simulink model "Block"  (R2017a)
settings: Solver=VariableStepAuto  StartTime=0.0  StopTime=Tsim  FixedStep=0.0001  RelTol=1e-3
values from neighbouring files (symbols this model uses):
  b = 0.1    [Model_old.m]
  g = 40    [Model_old.m]    (also in ModeloBase_OLD.m)
  J = 0.01    [Model_old.m]
  Kd = 0    [Model_old.m]
  Ke = 0.08    [Model_old.m]
  Ki = 10.0    (= 10)    [Model_old.m]
  Kp = 5.0    (= 5)    [Model_old.m]
  ksi = 0.6    [Model_old.m]    (also in ModeloBase_OLD.m = 0.3)
  L = 0.5    [Model_old.m]
  R = 1    [Model_old.m]
  Ts = 0.1    [Model_old.m]    (also in ModeloBase_OLD.m; PIController.m)
undefined symbols (not defined in the file or in its folder): DiscIntNeverNeededParam, F_M
libraries: simulink x16, simulink_extras x2
settings Model: Creator=davi2  LastModifiedBy=davi2

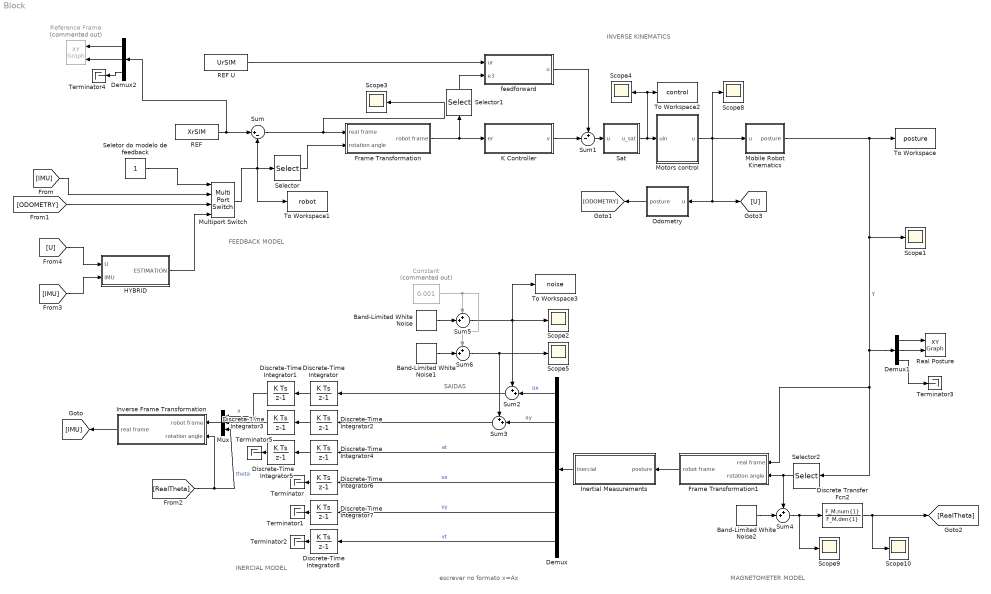
== system Block ==
  note: escrever no formato x=Ax
  note: SAIDAS
  note: INVERSE KINEMATICS
  note: MAGNETOMETER MODEL
  note: INERCIAL MODEL
  note: FEEDBACK MODEL
  Band-Limited White Noise : simulink/Sources/Band-Limited White Noise  Cov=0.000008  Ts=1/200  seed=[23341]
  Band-Limited White Noise1 : simulink/Sources/Band-Limited White Noise  Cov=0.000008  Ts=1/200  seed=[23341]
  Band-Limited White Noise2 : simulink/Sources/Band-Limited White Noise  Cov=0.00001  Ts=1/200  seed=[23341]
  Constant : Constant  Commented=on  Value=0.001
  Demux : Demux  Outputs=6
  Demux1 : Demux  Outputs=3
  Demux2 : Demux  Outputs=3
  Discrete Transfer Fcn2 : DiscreteTransferFcn  Numerator=F_M.num{1}  Denominator=F_M.den{1}
  Discrete-Time Integrator{,1..8} (9 alike) : DiscreteIntegrator  InitialConditionSetting=State (most efficient)  SampleTime=Ts  ICPrevOutput=DiscIntNeverNeededParam  ICPrevScaledInput=DiscIntNeverNeededParam
  Frame Transformation : Subsystem
  Frame Transformation1 : Subsystem
  HYBRID : Subsystem
  Inertial Measurements : Subsystem
  Inverse Frame Transformation : Subsystem
  K Controller : Subsystem
  Mobile Robot Kinematics : Subsystem
  Motors control : Subsystem
  Multiport Switch : MultiPortSwitch
  Mux : Mux  Inputs=3
  Odometry : Subsystem
  REF : FromWorkspace  VariableName=XrSIM  SampleTime=Ts  OutputAfterFinalValue=Holding final value
  REF U : FromWorkspace  VariableName=UrSIM  SampleTime=Ts  OutputAfterFinalValue=Holding final value
  Real Posture : simulink/Sinks/XY Graph  xmin=0  xmax=3  ymin=-0.8  ymax=1.5  st=Ts
  Reference Frame : simulink/Sinks/XY Graph  Commented=on  xmin=0  xmax=2  ymin=0  ymax=1.5  st=Ts
  Sat : Subsystem
  Scope{1..5,8..10} (8 alike) : Scope
  Selector : Selector  InputPortWidth=3  IndexOptions=Index vector (dialog)  Indices=3  OutputSizes=1
  Selector1 : Selector  InputPortWidth=3  IndexOptions=Index vector (dialog)  Indices=3  OutputSizes=1
  Selector2 : Selector  InputPortWidth=3  IndexOptions=Index vector (dialog)  Indices=3  OutputSizes=1
  Seletor do modelo de feedback : Constant
  Sum : Sum  Inputs=|+-
  Sum1 : Sum  Inputs=+-|
  Sum{2..6} (5 alike) : Sum  Inputs=++|
  Terminator{,1..5} (6 alike) : Terminator
  To Workspace : ToWorkspace  VariableName=posture  SaveFormat=Timeseries  SampleTime=-1
  To Workspace1 : ToWorkspace  VariableName=robot  SaveFormat=Timeseries  SampleTime=-1
  To Workspace2 : ToWorkspace  VariableName=control  SaveFormat=Timeseries  SampleTime=-1
  To Workspace3 : ToWorkspace  VariableName=noise  SaveFormat=Timeseries  SampleTime=-1
  feedforward : Subsystem
  wires:
  Sum/1 -> Scope3/1, Frame Transformation/1(real frame)
  Selector/1 -> Frame Transformation/2(rotation angle)
  Frame Transformation/1(robot frame) -> K Controller/1(er), Selector1/1
  REF U/1 -> feedforward/1(ur)
  Selector1/1 -> feedforward/2(e3)
  feedforward/1(u) -> Sum1/1
  K Controller/1(v) -> Sum1/2
  Motors control/1(u) -> Mobile Robot Kinematics/1(u), Scope8/1, Odometry/1(u), [U]
  Selector2/1 -> Frame Transformation1/2(rotation angle), Sum4/1
  Inertial Measurements/1(inercial) -> Demux/1
  Discrete-Time Integrator/1 -> Discrete-Time Integrator1/1
  Frame Transformation1/1(robot frame) -> Inertial Measurements/1(posture)
  Discrete-Time Integrator2/1 -> Discrete-Time Integrator3/1
  Discrete-Time Integrator4/1 -> Discrete-Time Integrator5/1
  Demux/4 -> Discrete-Time Integrator6/1  "vx"
  Demux/5 -> Discrete-Time Integrator7/1  "vy"
  Demux/6 -> Discrete-Time Integrator8/1  "vt"
  Discrete-Time Integrator1/1 -> Mux/1  "x"
  Discrete-Time Integrator3/1 -> Mux/2  "y"
  Mux/1 -> Inverse Frame Transformation/1(robot frame)
  Demux/1 -> Sum2/2  "ax"
  Demux1/1 -> Real Posture/1
  Demux1/2 -> Real Posture/2
  REF/1 -> Demux2/1, Sum/1
  Inverse Frame Transformation/1(real frame) -> [IMU]
  [IMU] -> Multiport Switch/2
  [ODOMETRY] -> Multiport Switch/3
  Odometry/1(posture) -> [ODOMETRY]
  Mobile Robot Kinematics/1(posture) -> To Workspace/1, Scope1/1, Demux1/1, Frame Transformation1/1(real frame), Selector2/1  "Y"
  Demux/3 -> Discrete-Time Integrator4/1  "at"
  Demux/2 -> Sum3/2  "ay"
  [RealTheta] -> Mux/3, Inverse Frame Transformation/2(rotation angle)  "theta"
  Sum2/1 -> Discrete-Time Integrator/1
  Sum3/1 -> Discrete-Time Integrator2/1
  Band-Limited White Noise/1 -> Sum5/2
  Sum5/1 -> To Workspace3/1, Scope2/1, Sum2/1
  Band-Limited White Noise1/1 -> Sum6/2
  Sum6/1 -> Scope5/1, Sum3/1
  Sum1/1 -> Sat/1(u)
  Sat/1(u_sat) -> Scope4/1, To Workspace2/1, Motors control/1(uin)
  Constant/1 -> Sum5/1, Sum6/1
  Multiport Switch/1 -> Sum/2, Selector/1, To Workspace1/1
  Discrete-Time Integrator6/1 -> Terminator/1
  Discrete-Time Integrator7/1 -> Terminator1/1
  Discrete-Time Integrator8/1 -> Terminator2/1
  Demux1/3 -> Terminator3/1
  Seletor do modelo de feedback/1 -> Multiport Switch/1
  Discrete-Time Integrator5/1 -> Terminator5/1
  HYBRID/1(ESTIMATION) -> Multiport Switch/4
  [IMU] -> HYBRID/2(IMU)
  [U] -> HYBRID/1(U)
  Band-Limited White Noise2/1 -> Sum4/2
  Sum4/1 -> Discrete Transfer Fcn2/1, Scope9/1
  Discrete Transfer Fcn2/1 -> [RealTheta], Scope10/1
  Demux2/1 -> Reference Frame/1
  Demux2/2 -> Reference Frame/2
  Demux2/3 -> Terminator4/1

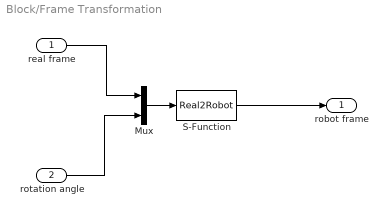
== system Block/Frame Transformation ==
  real frame : Inport
  rotation angle : Inport  Port=2
  Mux : Mux  Inputs=2
  S-Function : S-Function  FunctionName=Real2Robot  Parameters=Ts  SFunctionDeploymentMode=off  EnableBusSupport=off
  robot frame : Outport
  wires:
  real frame/1 -> Mux/1
  rotation angle/1 -> Mux/2
  Mux/1 -> S-Function/1
  S-Function/1 -> robot frame/1

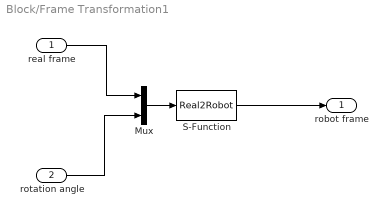
== system Block/Frame Transformation1 ==
  real frame : Inport
  rotation angle : Inport  Port=2
  Mux : Mux  Inputs=2
  S-Function : S-Function  FunctionName=Real2Robot  Parameters=Ts  SFunctionDeploymentMode=off  EnableBusSupport=off
  robot frame : Outport
  wires:
  real frame/1 -> Mux/1
  rotation angle/1 -> Mux/2
  Mux/1 -> S-Function/1
  S-Function/1 -> robot frame/1

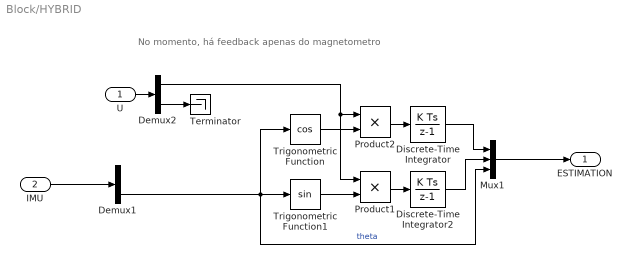
== system Block/HYBRID ==
  note: No momento, há feedback apenas do magnetometro
  U : Inport
  IMU : Inport  Port=2
  Demux1 : Demux  Outputs=3
  Demux2 : Demux  Outputs=2
  Discrete-Time Integrator : DiscreteIntegrator  InitialConditionSetting=State (most efficient)  SampleTime=Ts  ICPrevOutput=DiscIntNeverNeededParam  ICPrevScaledInput=DiscIntNeverNeededParam
  Discrete-Time Integrator2 : DiscreteIntegrator  InitialConditionSetting=State (most efficient)  SampleTime=Ts  ICPrevOutput=DiscIntNeverNeededParam  ICPrevScaledInput=DiscIntNeverNeededParam
  Mux1 : Mux  Inputs=3
  Product1 : Product
  Product2 : Product
  Terminator : Terminator
  Trigonometric Function : Trigonometry  Operator=cos
  Trigonometric Function1 : Trigonometry
  ESTIMATION : Outport
  wires:
  IMU/1 -> Demux1/1
  Trigonometric Function1/1 -> Product1/2
  Demux2/1 -> Product1/1, Product2/1
  Trigonometric Function/1 -> Product2/2
  Product2/1 -> Discrete-Time Integrator/1
  Discrete-Time Integrator/1 -> Mux1/1
  Discrete-Time Integrator2/1 -> Mux1/2
  Demux1/3 -> Mux1/3, Trigonometric Function/1, Trigonometric Function1/1  "theta"
  Product1/1 -> Discrete-Time Integrator2/1
  Mux1/1 -> ESTIMATION/1
  U/1 -> Demux2/1
  Demux2/2 -> Terminator/1

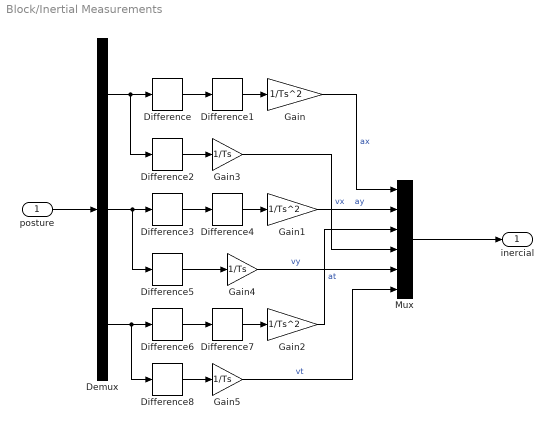
== system Block/Inertial Measurements ==
  posture : Inport
  Demux : Demux  Outputs=3
  Difference{,1..8} (9 alike) : simulink/Discrete/Difference  ICPrevInput=0.0  OutMin=[]  OutMax=[]  OutDataType=fixdt(1, 16)  OutScaling=2^-10  DoSatur=off
  Gain : Gain  Gain=1/Ts^2
  Gain1 : Gain  Gain=1/Ts^2
  Gain2 : Gain  Gain=1/Ts^2
  Gain3 : Gain  Gain=1/Ts
  Gain4 : Gain  Gain=1/Ts
  Gain5 : Gain  Gain=1/Ts
  Mux : Mux  Inputs=6
  inercial : Outport
  wires:
  posture/1 -> Demux/1
  Difference/1 -> Difference1/1
  Difference3/1 -> Difference4/1
  Difference6/1 -> Difference7/1
  Demux/3 -> Difference8/1, Difference6/1
  Demux/2 -> Difference5/1, Difference3/1
  Demux/1 -> Difference2/1, Difference/1
  Difference1/1 -> Gain/1
  Difference4/1 -> Gain1/1
  Difference7/1 -> Gain2/1
  Gain2/1 -> Mux/3  "at"
  Gain1/1 -> Mux/2  "ay"
  Gain/1 -> Mux/1  "ax"
  Difference2/1 -> Gain3/1
  Difference8/1 -> Gain5/1
  Difference5/1 -> Gain4/1
  Gain3/1 -> Mux/4  "vx"
  Gain4/1 -> Mux/5  "vy"
  Gain5/1 -> Mux/6  "vt"
  Mux/1 -> inercial/1

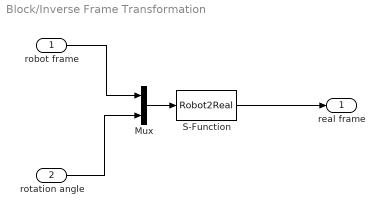
== system Block/Inverse Frame Transformation ==
  robot frame : Inport
  rotation angle : Inport  Port=2
  Mux : Mux  Inputs=2
  S-Function : S-Function  FunctionName=Robot2Real  Parameters=Ts  SFunctionDeploymentMode=off  EnableBusSupport=off
  real frame : Outport
  wires:
  robot frame/1 -> Mux/1
  rotation angle/1 -> Mux/2
  Mux/1 -> S-Function/1
  S-Function/1 -> real frame/1

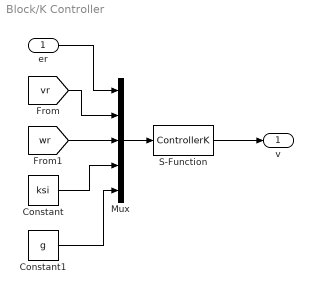
== system Block/K Controller ==
  er : Inport
  Constant : Constant  Value=ksi
  Constant1 : Constant  Value=g
  Mux : Mux  Inputs=5
  S-Function : S-Function  FunctionName=ControllerK  Parameters=Ts  SFunctionDeploymentMode=off  EnableBusSupport=off
  v : Outport
  wires:
  er/1 -> Mux/1
  [vr] -> Mux/2
  [wr] -> Mux/3
  Constant/1 -> Mux/4
  Constant1/1 -> Mux/5
  Mux/1 -> S-Function/1
  S-Function/1 -> v/1

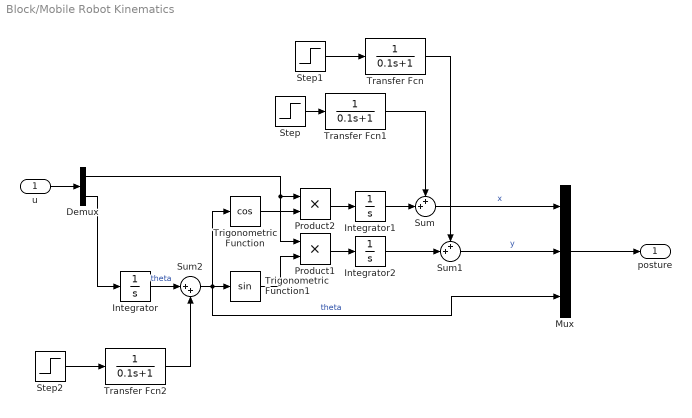
== system Block/Mobile Robot Kinematics ==
  u : Inport
  Demux : Demux  Outputs=2
  Integrator : Integrator
  Integrator1 : Integrator
  Integrator2 : Integrator
  Mux : Mux  Inputs=3
  Product1 : Product
  Product2 : Product
  Step : Step  Time=20  After=0.5  SampleTime=0
  Step1 : Step  Time=10  After=-0.5  SampleTime=0
  Step2 : Step  Time=5  After=0  SampleTime=0
  Sum : Sum  Inputs=++|
  Sum1 : Sum  Inputs=++|
  Sum2 : Sum  Inputs=|++
  Transfer Fcn : TransferFcn  Denominator=[0.1 1]
  Transfer Fcn1 : TransferFcn  Denominator=[0.1 1]
  Transfer Fcn2 : TransferFcn  Denominator=[0.1 1]
  Trigonometric Function : Trigonometry  Operator=cos
  Trigonometric Function1 : Trigonometry
  posture : Outport
  wires:
  u/1 -> Demux/1
  Demux/2 -> Integrator/1
  Trigonometric Function/1 -> Product2/2
  Demux/1 -> Product1/1, Product2/1
  Product2/1 -> Integrator1/1
  Trigonometric Function1/1 -> Product1/2
  Product1/1 -> Integrator2/1
  Mux/1 -> posture/1
  Transfer Fcn1/1 -> Sum/1
  Transfer Fcn/1 -> Sum1/1
  Step2/1 -> Transfer Fcn2/1
  Step1/1 -> Transfer Fcn/1
  Step/1 -> Transfer Fcn1/1
  Integrator1/1 -> Sum/2
  Integrator2/1 -> Sum1/2
  Sum/1 -> Mux/1  "x"
  Sum1/1 -> Mux/2  "y"
  Integrator/1 -> Sum2/1  "theta"
  Sum2/1 -> Trigonometric Function/1, Mux/3, Trigonometric Function1/1  "theta"
  Transfer Fcn2/1 -> Sum2/2

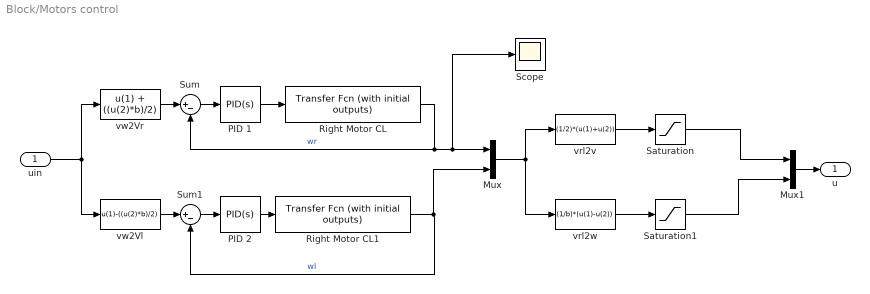
== system Block/Motors control ==
  uin : Inport
  Mux : Mux  Inputs=2
  Mux1 : Mux  Inputs=2
  PID 1 : simulink/Continuous/PID Controller  Controller=PID  TimeDomain=Continuous-time  SampleTime=-1  IntegratorMethod=Forward Euler  FilterMethod=Forward Euler  Form=Parallel  UseFilter=on  ControllerParametersSource=internal  P=Kp  I=Ki  D=Kd  N=100  InitialConditionSource=internal  InitialConditionForIntegrator=0  InitialConditionForFilter=0  ExternalReset=none  LimitOutput=off  UpperSaturationLimit=inf  LowerSaturationLimit=-inf  LinearizeAsGain=on  AntiWindupMode=none  Kb=1  TrackingMode=off  Kt=1  PParamMin=[]  PParamMax=[]  IParamMin=[]  IParamMax=[]  DParamMin=[]  DParamMax=[]  NParamMin=[]  NParamMax=[]  KbParamMin=[]  KbParamMax=[]  KtParamMin=[]  KtParamMax=[]  POutMin=[]  POutMax=[]  IOutMin=[]  IOutMax=[]  DOutMin=[]  DOutMax=[]  NOutMin=[]  NOutMax=[]  KbOutMin=[]  KbOutMax=[]  KtOutMin=[]  KtOutMax=[]  IntegratorOutMin=[]  IntegratorOutMax=[]  FilterOutMin=[]  FilterOutMax=[]  SumOutMin=[]  SumOutMax=[]  SumI1OutMin=[]  SumI1OutMax=[]  SumI2OutMin=[]  SumI2OutMax=[]  SumI3OutMin=[]  SumI3OutMax=[]  SumDOutMin=[]  SumDOutMax=[]  SaturationOutMin=[]  SaturationOutMax=[]  IntegratorContinuousStateAttributes=''  IntegratorStateMustResolveToSignalObject=off  IntegratorRTWStateStorageClass=Auto  FilterContinuousStateAttributes=''  FilterStateMustResolveToSignalObject=off  FilterRTWStateStorageClass=Auto  DifferentiatorICPrevScaledInput=0  DifferentiatorOutMin=[]  DifferentiatorOutMax=[]  InitialConditionSetting=State (most efficient)
  PID 2 : simulink/Continuous/PID Controller  Controller=PID  TimeDomain=Continuous-time  SampleTime=-1  IntegratorMethod=Forward Euler  FilterMethod=Forward Euler  Form=Parallel  UseFilter=on  ControllerParametersSource=internal  P=Kp  I=Ki  D=Kd  N=100  InitialConditionSource=internal  InitialConditionForIntegrator=0  InitialConditionForFilter=0  ExternalReset=none  LimitOutput=off  UpperSaturationLimit=inf  LowerSaturationLimit=-inf  LinearizeAsGain=on  AntiWindupMode=none  Kb=1  TrackingMode=off  Kt=1  PParamMin=[]  PParamMax=[]  IParamMin=[]  IParamMax=[]  DParamMin=[]  DParamMax=[]  NParamMin=[]  NParamMax=[]  KbParamMin=[]  KbParamMax=[]  KtParamMin=[]  KtParamMax=[]  POutMin=[]  POutMax=[]  IOutMin=[]  IOutMax=[]  DOutMin=[]  DOutMax=[]  NOutMin=[]  NOutMax=[]  KbOutMin=[]  KbOutMax=[]  KtOutMin=[]  KtOutMax=[]  IntegratorOutMin=[]  IntegratorOutMax=[]  FilterOutMin=[]  FilterOutMax=[]  SumOutMin=[]  SumOutMax=[]  SumI1OutMin=[]  SumI1OutMax=[]  SumI2OutMin=[]  SumI2OutMax=[]  SumI3OutMin=[]  SumI3OutMax=[]  SumDOutMin=[]  SumDOutMax=[]  SaturationOutMin=[]  SaturationOutMax=[]  IntegratorContinuousStateAttributes=''  IntegratorStateMustResolveToSignalObject=off  IntegratorRTWStateStorageClass=Auto  FilterContinuousStateAttributes=''  FilterStateMustResolveToSignalObject=off  FilterRTWStateStorageClass=Auto  DifferentiatorICPrevScaledInput=0  DifferentiatorOutMin=[]  DifferentiatorOutMax=[]  InitialConditionSetting=State (most efficient)
  Right Motor CL : simulink_extras/Additional Linear/Transfer Fcn (with initial outputs)  N=[Ke]  D="[J*L  (J*R+b*L) (b*R+Ke^2)]"  Y0=0  U0=0
  Right Motor CL1 : simulink_extras/Additional Linear/Transfer Fcn (with initial outputs)  N=[Ke]  D="[J*L  (J*R+b*L) (b*R+Ke^2)]"  Y0=0  U0=0
  Saturation : Saturate  UpperLimit=1  LowerLimit=-1
  Saturation1 : Saturate  UpperLimit=1  LowerLimit=-1
  Scope : Scope
  Sum : Sum  Inputs=|+-
  Sum1 : Sum  Inputs=|+-
  vrl2v : Fcn  Expr=(1/2)*(u(1)+u(2))
  vrl2w : Fcn  Expr=(1/b)*(u(1)-u(2))
  vw2Vl : Fcn  Expr=u(1)-((u(2)*b)/2)
  vw2Vr : Fcn  Expr=u(1) + ((u(2)*b)/2)
  u : Outport
  wires:
  vw2Vr/1 -> Sum/1
  Right Motor CL1/1 -> Mux/2, Sum1/2  "wl"
  vw2Vl/1 -> Sum1/1
  Sum1/1 -> PID 2/1
  PID 2/1 -> Right Motor CL1/1
  Sum/1 -> PID 1/1
  PID 1/1 -> Right Motor CL/1
  Right Motor CL/1 -> Mux/1, Scope/1, Sum/2  "wr"
  uin/1 -> vw2Vl/1, vw2Vr/1
  Mux/1 -> vrl2v/1, vrl2w/1
  Mux1/1 -> u/1
  vrl2w/1 -> Saturation1/1
  vrl2v/1 -> Saturation/1
  Saturation/1 -> Mux1/1
  Saturation1/1 -> Mux1/2

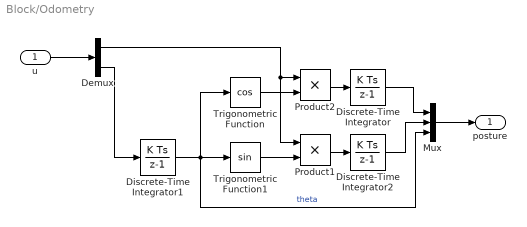
== system Block/Odometry ==
  u : Inport
  Demux : Demux  Outputs=2
  Discrete-Time Integrator : DiscreteIntegrator  InitialConditionSetting=State (most efficient)  SampleTime=Ts  ICPrevOutput=DiscIntNeverNeededParam  ICPrevScaledInput=DiscIntNeverNeededParam
  Discrete-Time Integrator1 : DiscreteIntegrator  InitialConditionSetting=State (most efficient)  SampleTime=Ts  ICPrevOutput=DiscIntNeverNeededParam  ICPrevScaledInput=DiscIntNeverNeededParam
  Discrete-Time Integrator2 : DiscreteIntegrator  InitialConditionSetting=State (most efficient)  SampleTime=Ts  ICPrevOutput=DiscIntNeverNeededParam  ICPrevScaledInput=DiscIntNeverNeededParam
  Mux : Mux  Inputs=3
  Product1 : Product
  Product2 : Product
  Trigonometric Function : Trigonometry  Operator=cos
  Trigonometric Function1 : Trigonometry
  posture : Outport
  wires:
  u/1 -> Demux/1
  Demux/2 -> Discrete-Time Integrator1/1
  Discrete-Time Integrator1/1 -> Mux/3, Trigonometric Function/1, Trigonometric Function1/1  "theta"
  Trigonometric Function/1 -> Product2/2
  Demux/1 -> Product1/1, Product2/1
  Product2/1 -> Discrete-Time Integrator/1
  Trigonometric Function1/1 -> Product1/2
  Product1/1 -> Discrete-Time Integrator2/1
  Discrete-Time Integrator/1 -> Mux/1
  Discrete-Time Integrator2/1 -> Mux/2
  Mux/1 -> posture/1

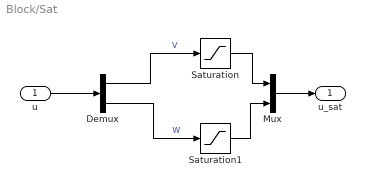
== system Block/Sat ==
  u : Inport
  Demux : Demux  Outputs=2
  Mux : Mux  Inputs=2
  Saturation : Saturate  LowerLimit=0
  Saturation1 : Saturate
  u_sat : Outport
  wires:
  Demux/2 -> Saturation1/1  "W"
  Demux/1 -> Saturation/1  "V"
  u/1 -> Demux/1
  Saturation/1 -> Mux/1
  Saturation1/1 -> Mux/2
  Mux/1 -> u_sat/1

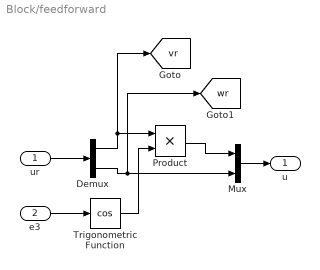
== system Block/feedforward ==
  ur : Inport
  e3 : Inport  Port=2
  Demux : Demux  Outputs=2
  Mux : Mux  Inputs=2
  Product : Product
  Trigonometric Function : Trigonometry  Operator=cos
  u : Outport
  tag scope: vr=global, wr=global
  wires:
  e3/1 -> Trigonometric Function/1
  ur/1 -> Demux/1
  Demux/1 -> [vr], Product/1
  Trigonometric Function/1 -> Product/2
  Product/1 -> Mux/1
  Demux/2 -> [wr], Mux/2
  Mux/1 -> u/1
